simulink model "Simulink_Lab2"  (R2022b)
settings: Solver=VariableStepAuto  StartTime=0.0  StopTime=10.0  RelTol=1e-3
settings Model: Creator=ahmed  LastModifiedBy=ahmed

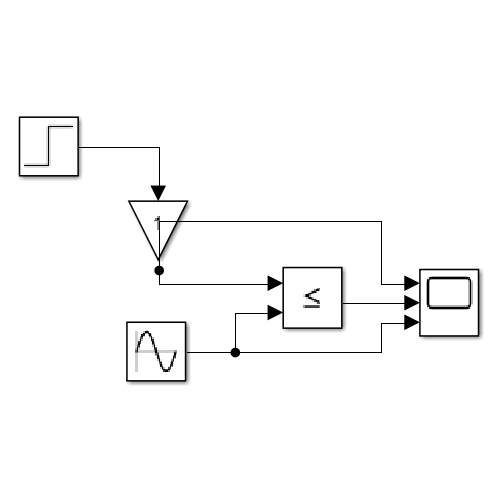
[thumbnail: Simulink's stored preview of the top-level diagram]
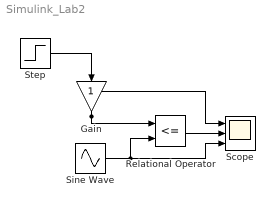
== system Simulink_Lab2 ==
  Gain : Gain
  Relational Operator : RelationalOperator  Operator=<=  OutDataTypeStr=boolean  RndMeth=Simplest  InputSameDT=off
  Scope : Scope  NumInputPorts=3
  Sine Wave : Sin  SampleTime=0
  Step : Step  Time=2  SampleTime=0
  wires:
  Step/1 -> Gain/1
  Gain/1 -> Relational Operator/1, Scope/1
  Relational Operator/1 -> Scope/2
  Sine Wave/1 -> Scope/3, Relational Operator/2
